simulink model "for_decomposition"  (R2020a)
settings: Solver=VariableStepAuto  StartTime=0.0  StopTime=10.0  RelTol=1e-3
model workspace (MAT data in the model file):
  K = 0.00399
  T11 = 0.1738
  T12 = 144.88
  T21 = 2.04e-05
  T22 = 0.0511
  T23 = 0.1899
settings Model: OrderedModelArguments=off  Creator=Sainquake  LastModifiedBy=Sainquake

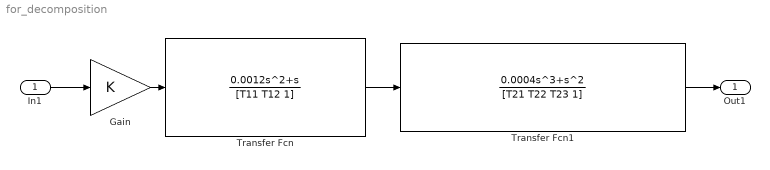
== system for_decomposition ==
  In1 : Inport
  Gain : Gain  Gain=K
  Transfer Fcn : TransferFcn  Numerator=[0.0012 1 0]  Denominator=[T11 T12 1]
  Transfer Fcn1 : TransferFcn  Numerator=[0.0004 1 0 0]  Denominator=[T21 T22 T23 1]
  Out1 : Outport
  wires:
  Transfer Fcn/1 -> Transfer Fcn1/1
  Transfer Fcn1/1 -> Out1/1
  In1/1 -> Gain/1
  Gain/1 -> Transfer Fcn/1
